simulink model "sl_subsys_fcncallerr5"  (Simulink 6.0)
settings: Solver=FixedStepDiscrete  StartTime=0.0  StopTime=10.0  FixedStep=1  RelTol=1e-3
settings Model: CovMetricSettings=d  Creator=The MathWorks Inc.  LastModifiedBy=batserve  ExtModeAutoUpdateStatusClock=off
settings OptimizationCC: BlockReduction=off  BooleanDataType=off
settings DebuggingCC: CheckExecutionContextPreStartOutputMsg=on  CheckExecutionContextRuntimeOutputMsg=on  SolverPrmCheckMsg=none
settings HardwareCC: TargetUnknown=on

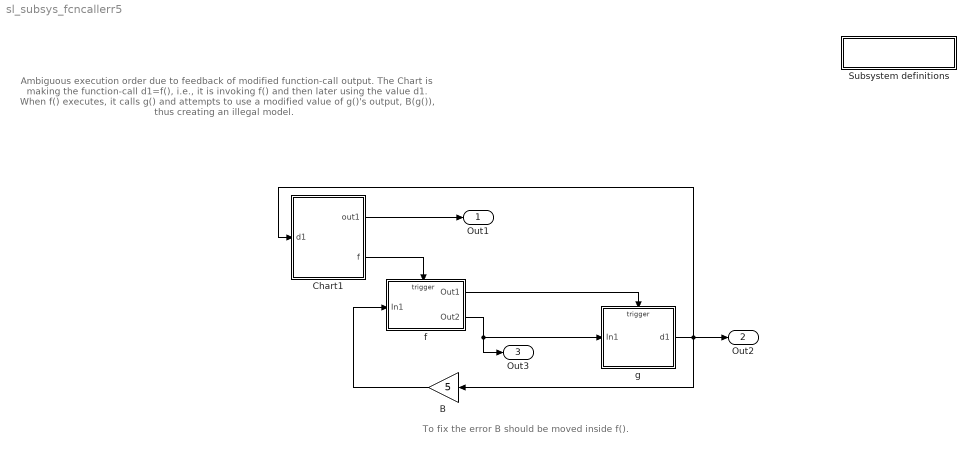
== system sl_subsys_fcncallerr5 ==
  note: Ambiguous execution order due to feedback of modified function-call output.
      |
      | The Chart is making the function-call d1=f(), i.e., it is invoking f() and then
      | later using the value d1. When f() executes, it calls g() and attempts to use a
      | modified value of g()'s output, B(g()), thus creating an illegal model.
  note: To fix the error B should be moved inside f().
  " Subsystem definitions" : Subsystem  PropExecContextAcrossSSBoundary=on
      settings: OpenFcn=helpview([matlabroot,'/toolbox/simulink/simdemos/sl_subsys_definitions.html']);
      mask Display: disp('Subsystem\ndefinitions')
  B : Gain  Orientation=left  Gain=5  SaturateOnIntegerOverflow=on
  Chart1 : Stateflow chart  PropExecContextAcrossSSBoundary=on
  f : Subsystem  TreatAsAtomicUnit=on  PropExecContextAcrossSSBoundary=on
  g : Subsystem  TreatAsAtomicUnit=on  PropExecContextAcrossSSBoundary=on
  Out1 : Outport
  Out2 : Outport  Port=2
  Out3 : Outport  Port=3
  wires:
  Chart1/2(f) -> f/Trigger
  f/1(Out1) -> g/Trigger
  f/2(Out2) -> Out3/1, g/1(In1)
  g/1(d1) -> Out2/1, B/1, Chart1/1(d1)
  Chart1/1(out1) -> Out1/1
  B/1 -> f/1(In1)

== system sl_subsys_fcncallerr5/ Subsystem definitions ==

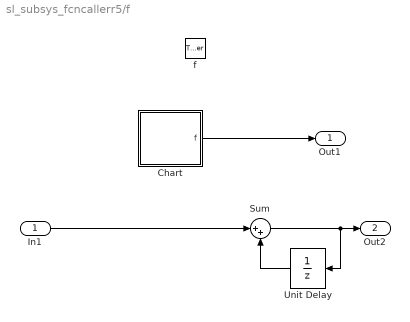
== system sl_subsys_fcncallerr5/f ==
  In1 : Inport  Port=1  LatchInput=off
  f : TriggerPort  TriggerType=function-call
  Chart : Stateflow chart  PropExecContextAcrossSSBoundary=on
  Sum : Sum  Inputs=|++  SaturateOnIntegerOverflow=on  InputSameDT=on
  Unit Delay : UnitDelay  Orientation=left  SampleTime=-1
  Out1 : Outport
  Out2 : Outport  Port=2
  wires:
  Chart/1(f) -> Out1/1
  In1/1 -> Sum/1
  Unit Delay/1 -> Sum/2
  Sum/1 -> Out2/1, Unit Delay/1

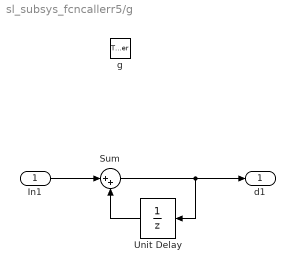
== system sl_subsys_fcncallerr5/g ==
  In1 : Inport  Port=1  LatchInput=off
  g : TriggerPort  TriggerType=function-call
  Sum : Sum  Inputs=|++  SaturateOnIntegerOverflow=on  InputSameDT=on
  Unit Delay : UnitDelay  Orientation=left  SampleTime=-1
  d1 : Outport
  wires:
  In1/1 -> Sum/1
  Unit Delay/1 -> Sum/2
  Sum/1 -> d1/1, Unit Delay/1

== stateflow chart f/Chart ==
  state one
  state two
  one -> two : /f;
  two -> one : /f;
  (default) -> one
  events: f output FUNCTION_CALL_EVENT

== stateflow chart Chart1 ==
  state one/
    entry:f;out1=d1+5;
  state two/
    entry: f;out1=d1-5;
  one -> two
  two -> one
  (default) -> one
  data: d1 input double; out1 output double; out local double
  events: f output FUNCTION_CALL_EVENT
